simulink model "full_maneuver_platoon_new_strategy"  (R2019a)
settings: Solver=VariableStepAuto  StartTime=0.0  StopTime=70  FixedStep=0.1  MaxStep=0.05  RelTol=1e-3
libraries: simulink x97, dspsigops x7, powerlib_meascontrol x7, autolibshared x7
(part 3 of 7)

== system full_maneuver_platoon_new_strategy/Fd/safeErrors ==
  errors : Inport
  AND : Logic  IconShape=distinctive  AllPortsSameDT=off  OutDataTypeStr=boolean
  Compare To Constant4 : simulink/Logic and Bit Operations/Compare To Constant  relop=>=  const=-0.1  OutDataTypeStr=boolean
  Demux : Demux  Outputs=2
  safetyFlag : Outport
  wires:
  Demux/2 -> AND/2
  Demux/1 -> AND/1
  AND/1 -> safetyFlag/1
  errors/1 -> Compare To Constant4/1
  Compare To Constant4/1 -> Demux/1

== system full_maneuver_platoon_new_strategy/Fd/safeErrors1 ==
  errors : Inport
  AND : Logic  IconShape=distinctive  AllPortsSameDT=off  OutDataTypeStr=boolean
  Compare To Constant4 : simulink/Logic and Bit Operations/Compare To Constant  relop=>=  const=-0.1  OutDataTypeStr=boolean
  Demux : Demux  Outputs=2
  safetyFlag : Outport
  wires:
  Compare To Constant4/1 -> Demux/1
  errors/1 -> Compare To Constant4/1
  AND/1 -> safetyFlag/1
  Demux/1 -> AND/1
  Demux/2 -> AND/2

== system full_maneuver_platoon_new_strategy/Fd/safeErrors2 ==
  errors : Inport
  AND : Logic  IconShape=distinctive  AllPortsSameDT=off  OutDataTypeStr=boolean
  Compare To Constant4 : simulink/Logic and Bit Operations/Compare To Constant  relop=>=  const=-0.1  OutDataTypeStr=boolean
  Demux : Demux  Outputs=2
  safetyFlag : Outport
  wires:
  Demux/2 -> AND/2
  Demux/1 -> AND/1
  AND/1 -> safetyFlag/1
  errors/1 -> Compare To Constant4/1
  Compare To Constant4/1 -> Demux/1

== system full_maneuver_platoon_new_strategy/Fd/steadyState ==
  u : Inport
  AND : Logic  IconShape=distinctive  AllPortsSameDT=off  OutDataTypeStr=boolean
  Abs2 : Abs
  Compare To Constant2 : simulink/Logic and Bit Operations/Compare To Constant  relop=<=  const=0.2  OutDataTypeStr=boolean
  Demux : Demux  Outputs=2
  Mux : Mux  Inputs=2
  Transport Delay2 : TransportDelay
  ssFlag : Outport
  wires:
  u/1 -> Transport Delay2/1, Mux/2
  Abs2/1 -> Compare To Constant2/1
  Demux/1 -> AND/1
  Transport Delay2/1 -> Mux/1
  AND/1 -> ssFlag/1
  Compare To Constant2/1 -> Demux/1
  Mux/1 -> Abs2/1
  Demux/2 -> AND/2

== system full_maneuver_platoon_new_strategy/Fo/Lateral Control ==
  <Y> : Inport
  <r> : Inport  Port=2
  startLaneChange : Inport  Port=3
  yRef : Inport  Port=4
  Demux2 : Demux
  Full State Observer : Subsystem
  Gain1 : Gain  Gain=Klat  Multiplication=Matrix(K*u)
  Integrator : Integrator  InitialCondition=y0
  Mux : Mux  Inputs=2
  Pad : dspsigops/Pad  padAlong=Columns  dimsToPad=1  valSrc=Specify via dialog  padVal=0  spec=Output size  padNumOutRowsSpecMethod=User-specified  numOutRows=4  padNumOutColsSpecMethod=User-specified  numOutCols=1  isVarDimsMode=off  padBeginning=0  padEnd=0  outSizeMode=User-specified  outSize=1  padSigAt=End  trunc_flag=None  roundingMode=Floor  overflowMode=off  truncOrWrapMode=Truncate  wrap_flag=None
      settings: SourceProductName=DSP System Toolbox  SourceProductBaseCode=DS
  Rate Limiter : RateLimiter  RisingSlewLimit=maxDeltaDot  FallingSlewLimit=-maxDeltaDot  SampleTimeMode=inherited
  Saturation : Saturate  UpperLimit=maxDelta  LowerLimit=-maxDelta
  Scope : Scope  NumInputPorts=4
  Scope1 : Scope
  Sum : Sum  Inputs=|+-
  Sum2 : Sum  Inputs=|+-
  Triggered Subsystem1 : Subsystem  TreatAsAtomicUnit=on
  delta : Outport
  wires:
  Rate Limiter/1 -> Full State Observer/2(delta), Scope1/1, delta/1  "delta"
  Demux2/1 -> Scope/1
  Integrator/1 -> Sum2/2, Pad/1
  Gain1/1 -> Saturation/1
  <r>/1 -> Mux/2
  Full State Observer/1(xhat) -> Sum/2, Demux2/1  "estStates"
  Sum/1 -> Gain1/1
  Pad/1 -> Sum/1
  Mux/1 -> Full State Observer/1(measuredOutputs)
  Demux2/4 -> Scope/4
  Demux2/2 -> Scope/2
  Sum2/1 -> Integrator/1
  Saturation/1 -> Rate Limiter/1
  Demux2/3 -> Scope/3
  Triggered Subsystem1/1(Out1) -> Sum2/1
  <Y>/1 -> Mux/1
  startLaneChange/1 -> Triggered Subsystem1/Trigger
  yRef/1 -> Triggered Subsystem1/1(In1)

== system full_maneuver_platoon_new_strategy/Fo/Regular Vehicle Following ==
  ego : Inport
  leader : Inport  Port=2
  lcFlag : Inport  Port=3
  Bus Selector : BusSelector  OutputSignals=X,Xdot,u
  Bus Selector1 : BusSelector  OutputSignals=X,Xdot
  Chart : Stateflow chart  BlockKeywords=__PRM__SERIALIZED__DATA__:Stateflow Chart,Stateflow Diagram  TreatAsAtomicUnit=on
  Compare To Constant : simulink/Logic and Bit Operations/Compare To Constant  relop=<  const=5*maxHeadwayError  OutDataTypeStr=boolean
  Compute Errors : Subsystem
  Mux : Mux  Inputs=2
  Rate Limiter : RateLimiter  RisingSlewLimit=maxJerk  FallingSlewLimit=minJerk  SampleTimeMode=inherited
  Rate Limiter1 : RateLimiter  RisingSlewLimit=maxComfJerk  FallingSlewLimit=minComfJerk  SampleTimeMode=inherited
  Scope2 : Scope
  Scope3 : Scope
  Switch1 : Switch  Criteria=u2 > Threshold
  Veh Following : Subsystem  TreatAsAtomicUnit=on
  Velocity Control : Subsystem  TreatAsAtomicUnit=on
  comf saturation : Saturate  UpperLimit=maxComfAccel  LowerLimit=minComfAccel
  safe saturation : Saturate  UpperLimit=maxAcceleration  LowerLimit=minAcceleration
  veh foll state : Scope
  u : Outport
  errors : Outport  Port=2
  gap : Outport  Port=3
  wires:
  Bus Selector/2 -> Compute Errors/2(vf), Velocity Control/1(velocity)  "<Xdot>"
  Bus Selector/1 -> Compute Errors/1(xf)  "<X>"
  Veh Following/1(u) -> Chart/2(uVehFoll)
  lcFlag/1 -> Compute Errors/5(lcFlag)
  Compute Errors/1(eh) -> Compare To Constant/1, Veh Following/1(eh), Mux/1
  Compare To Constant/1 -> Chart/1(leaderWithinRange), Veh Following/4(intReset), Velocity Control/3(intReset)
  ego/1 -> Bus Selector/1
  Compute Errors/3("gap ") -> gap/1
  Compute Errors/4(unsafeFlag) -> Switch1/2, Scope2/1
  Rate Limiter1/1 -> Switch1/3  "sat(u)"
  Bus Selector/3 -> Veh Following/3(realInput), Velocity Control/2(realInput)  "<u>"
  Chart/2(u) -> safe saturation/1, comf saturation/1
  Switch1/1 -> u/1, Scope3/1
  Rate Limiter/1 -> Switch1/1  "sat(u)"
  safe saturation/1 -> Rate Limiter/1
  comf saturation/1 -> Rate Limiter1/1
  Compute Errors/2(ev) -> Veh Following/2(ev), Mux/2
  Velocity Control/1(u) -> Chart/3(uVelControl)
  Bus Selector1/1 -> Compute Errors/3(xl)  "<X>"
  Mux/1 -> errors/1
  Chart/1(state) -> veh foll state/1
  leader/1 -> Bus Selector1/1
  Bus Selector1/2 -> Compute Errors/4(vl)  "<Xdot>"

== system full_maneuver_platoon_new_strategy/Fo/Triggered Subsystem ==
  Trigger : TriggerPort  VariantControl=Variant
  Constant : Constant
  Out1 : Outport  InitialOutput=0
  wires:
  Constant/1 -> Out1/1

== system full_maneuver_platoon_new_strategy/Fo/Vehicle Following During LC ==
  ego : Inport
  futureLeader : Inport  Port=2
  lcFlag : Inport  Port=3
  Enable : EnablePort
  Bus Selector : BusSelector  OutputSignals=X,Xdot,u
  Bus Selector1 : BusSelector  OutputSignals=X,Xdot
  Chart : Stateflow chart  BlockKeywords=__PRM__SERIALIZED__DATA__:Stateflow Chart,Stateflow Diagram  TreatAsAtomicUnit=on
  Compare To Constant : simulink/Logic and Bit Operations/Compare To Constant  relop=<  const=5*maxHeadwayError  OutDataTypeStr=boolean
  Compute Errors : Subsystem
  Mux : Mux  Inputs=2
  Rate Limiter : RateLimiter  RisingSlewLimit=maxJerk  FallingSlewLimit=minJerk  SampleTimeMode=inherited
  Scope3 : Scope
  Subsystem : Subsystem
  Terminator : Terminator
  Veh Following : Subsystem  TreatAsAtomicUnit=on
  Velocity Control : Subsystem  TreatAsAtomicUnit=on
  safe saturation : Saturate  UpperLimit=maxAcceleration  LowerLimit=minAcceleration
  veh foll state : Scope
  u : Outport
  errors : Outport  Port=2
  gap : Outport  Port=3
  lcDone : Outport  Port=4
  wires:
  futureLeader/1 -> Bus Selector1/1, Subsystem/2(futureLeader)
  Subsystem/1(lcDone) -> lcDone/1
  Bus Selector/2 -> Velocity Control/1(velocity), Compute Errors/2(vf)  "<Xdot>"
  Compute Errors/1(eh) -> Mux/1, Veh Following/1(eh), Compare To Constant/1
  Compute Errors/4(unsafeFlag) -> Terminator/1
  Chart/1(state) -> veh foll state/1
  Compute Errors/2(ev) -> Veh Following/2(ev), Mux/2
  Bus Selector1/1 -> Compute Errors/3(xl)  "<X>"
  Mux/1 -> errors/1
  lcFlag/1 -> Compute Errors/5(lcFlag), Subsystem/3(lcFlag)
  Bus Selector/3 -> Velocity Control/2(realInput), Veh Following/3(realInput)  "<u>"
  Rate Limiter/1 -> Scope3/1, u/1  "sat(u)"
  safe saturation/1 -> Rate Limiter/1
  Chart/2(u) -> safe saturation/1
  Velocity Control/1(u) -> Chart/3(uVelControl)
  ego/1 -> Subsystem/1(ego), Bus Selector/1
  Veh Following/1(u) -> Chart/2(uVehFoll)
  Compare To Constant/1 -> Velocity Control/3(intReset), Veh Following/4(intReset), Chart/1(leaderWithinRange)
  Bus Selector/1 -> Compute Errors/1(xf)  "<X>"
  Compute Errors/3("gap ") -> gap/1
  Bus Selector1/2 -> Compute Errors/4(vl)  "<Xdot>"

== system full_maneuver_platoon_new_strategy/Fo/Virtual Vehicle Following ==
  ego : Inport
  virtualLeader : Inport  Port=2
  lcFlag : Inport  Port=3
  Enable : EnablePort
  Bus Selector : BusSelector  OutputSignals=X,Xdot,u
  Bus Selector1 : BusSelector  OutputSignals=X,Xdot
  Chart : Stateflow chart  BlockKeywords=__PRM__SERIALIZED__DATA__:Stateflow Chart,Stateflow Diagram  TreatAsAtomicUnit=on
  Compute Errors : Subsystem
  Input Saturation : Saturate  UpperLimit=maxComfAccel  LowerLimit=minComfAccel
  Mux : Mux  Inputs=2
  Rate Limiter : RateLimiter  RisingSlewLimit=maxComfJerk  FallingSlewLimit=minComfJerk  SampleTimeMode=inherited
  Subsystem : Subsystem
  Sum6 : Sum  Inputs=|+-
  Terminator : Terminator
  Transport Delay1 : TransportDelay  DelayTime=0.01
  Velocity Control : Subsystem  TreatAsAtomicUnit=on
  Virtual Leader Following : Subsystem  TreatAsAtomicUnit=on
  vMin : Constant  Value=vMin
  u : Outport  InitialOutput=0
  virtualErrors : Outport  Port=2  OutputWhenDisabled=reset  InitialOutput=[0, 0]
  virtualGap : Outport  Port=3  OutputWhenDisabled=reset  InitialOutput=[0]
  lcStarted : Outport  Port=4
  wires:
  Subsystem/1(lcStarted) -> lcStarted/1
  Sum6/1 -> Velocity Control/2(ev), Chart/1(velDiff)
  virtualLeader/1 -> Subsystem/2(virtualLeader), Bus Selector1/1
  Rate Limiter/1 -> u/1  "virtualFoll"
  Mux/1 -> virtualErrors/1
  vMin/1 -> Sum6/1
  Compute Errors/1(eh) -> Virtual Leader Following/1(eh), Mux/1  "eh"
  Bus Selector/3 -> Virtual Leader Following/3(realInput)  "<u>"
  ego/1 -> Subsystem/1(ego), Bus Selector/1
  Transport Delay1/1 -> Velocity Control/1(intReset)
  Virtual Leader Following/1(u) -> Chart/3(uVehFoll)  "uVehFoll"
  Bus Selector/2 -> Compute Errors/2(vf), Sum6/2  "<Xdot>"
  Input Saturation/1 -> Rate Limiter/1
  Bus Selector/1 -> Compute Errors/1(xf)  "<X>"
  Compute Errors/3("gap ") -> virtualGap/1
  Chart/2(u) -> Input Saturation/1  "u"
  Compute Errors/4(unsafeFlag) -> Terminator/1
  Chart/1(state) -> Transport Delay1/1
  Bus Selector1/1 -> Compute Errors/3(xl)  "<X>"
  Velocity Control/1(Out1) -> Chart/2(uVelControl)  "uVelControl"
  Compute Errors/2(ev) -> Mux/2, Virtual Leader Following/2(ev)
  lcFlag/1 -> Compute Errors/5(lcFlag)
  Bus Selector1/2 -> Compute Errors/4(vl)  "<Xdot>"

== system full_maneuver_platoon_new_strategy/Fo/followerErrors ==
  ego : Inport
  follower : Inport  Port=2
  Bus Selector1 : BusSelector  OutputSignals=X,Xdot
  Bus Selector3 : BusSelector  OutputSignals=X,Xdot
  Mux : Mux  Inputs=2
  Sum3 : Sum  Inputs=-+|
  Terminator1 : Terminator
  gapToFollower : Subsystem
  errors : Outport
  wires:
  gapToFollower/2("gap ") -> Terminator1/1
  Sum3/1 -> Mux/2
  Bus Selector3/2 -> gapToFollower/2(vf), Sum3/1  "<Xdot>"
  follower/1 -> Bus Selector3/1
  gapToFollower/1(eh) -> Mux/1
  Bus Selector1/2 -> Sum3/2  "<Xdot>"
  Bus Selector3/1 -> gapToFollower/1(xf)  "<X>"
  ego/1 -> Bus Selector1/1
  Bus Selector1/1 -> gapToFollower/3(xl)  "<X>"
  Mux/1 -> errors/1

== system full_maneuver_platoon_new_strategy/Fo/safeErrors ==
  errors : Inport
  AND : Logic  IconShape=distinctive  AllPortsSameDT=off  OutDataTypeStr=boolean
  Compare To Constant4 : simulink/Logic and Bit Operations/Compare To Constant  relop=>=  const=-0.1  OutDataTypeStr=boolean
  Demux : Demux  Outputs=2
  safetyFlag : Outport
  wires:
  Demux/2 -> AND/2
  Demux/1 -> AND/1
  AND/1 -> safetyFlag/1
  errors/1 -> Compare To Constant4/1
  Compare To Constant4/1 -> Demux/1

== system full_maneuver_platoon_new_strategy/Fo/safeErrors1 ==
  errors : Inport
  AND : Logic  IconShape=distinctive  AllPortsSameDT=off  OutDataTypeStr=boolean
  Compare To Constant4 : simulink/Logic and Bit Operations/Compare To Constant  relop=>=  const=-0.1  OutDataTypeStr=boolean
  Demux : Demux  Outputs=2
  safetyFlag : Outport
  wires:
  Compare To Constant4/1 -> Demux/1
  errors/1 -> Compare To Constant4/1
  AND/1 -> safetyFlag/1
  Demux/1 -> AND/1
  Demux/2 -> AND/2

== system full_maneuver_platoon_new_strategy/Fo/safeErrors2 ==
  errors : Inport
  AND : Logic  IconShape=distinctive  AllPortsSameDT=off  OutDataTypeStr=boolean
  Compare To Constant4 : simulink/Logic and Bit Operations/Compare To Constant  relop=>=  const=-0.1  OutDataTypeStr=boolean
  Demux : Demux  Outputs=2
  safetyFlag : Outport
  wires:
  Demux/2 -> AND/2
  Demux/1 -> AND/1
  AND/1 -> safetyFlag/1
  errors/1 -> Compare To Constant4/1
  Compare To Constant4/1 -> Demux/1

== system full_maneuver_platoon_new_strategy/Fo/steadyState ==
  u : Inport
  AND : Logic  IconShape=distinctive  AllPortsSameDT=off  OutDataTypeStr=boolean
  Abs1 : Abs
  Abs2 : Abs
  Compare To Constant1 : simulink/Logic and Bit Operations/Compare To Constant  relop=<=  const=0.5  OutDataTypeStr=boolean
  Compare To Constant2 : simulink/Logic and Bit Operations/Compare To Constant  relop=<=  const=0.5  OutDataTypeStr=boolean
  Transport Delay2 : TransportDelay
  ssFlag : Outport
  wires:
  u/1 -> Abs2/1, Transport Delay2/1
  Abs1/1 -> Compare To Constant1/1
  Abs2/1 -> Compare To Constant2/1
  Compare To Constant1/1 -> AND/1
  Transport Delay2/1 -> Abs1/1
  AND/1 -> ssFlag/1
  Compare To Constant2/1 -> AND/2

== system full_maneuver_platoon_new_strategy/Ld/Lateral Control ==
  <Y> : Inport
  <r> : Inport  Port=2
  startLaneChange : Inport  Port=3
  yRef : Inport  Port=4
  Demux2 : Demux
  Full State Observer : Subsystem
  Gain1 : Gain  Gain=Klat  Multiplication=Matrix(K*u)
  Integrator : Integrator  InitialCondition=y0
  Mux : Mux  Inputs=2
  Pad : dspsigops/Pad  padAlong=Columns  dimsToPad=1  valSrc=Specify via dialog  padVal=0  spec=Output size  padNumOutRowsSpecMethod=User-specified  numOutRows=4  padNumOutColsSpecMethod=User-specified  numOutCols=1  isVarDimsMode=off  padBeginning=0  padEnd=0  outSizeMode=User-specified  outSize=1  padSigAt=End  trunc_flag=None  roundingMode=Floor  overflowMode=off  truncOrWrapMode=Truncate  wrap_flag=None
      settings: SourceProductName=DSP System Toolbox  SourceProductBaseCode=DS
  Rate Limiter : RateLimiter  RisingSlewLimit=maxDeltaDot  FallingSlewLimit=-maxDeltaDot  SampleTimeMode=inherited
  Saturation : Saturate  UpperLimit=maxDelta  LowerLimit=-maxDelta
  Scope : Scope  NumInputPorts=4
  Scope1 : Scope
  Sum : Sum  Inputs=|+-
  Sum2 : Sum  Inputs=|+-
  Triggered Subsystem1 : Subsystem  TreatAsAtomicUnit=on
  delta : Outport
  wires:
  Rate Limiter/1 -> Full State Observer/2(delta), Scope1/1, delta/1  "delta"
  Demux2/1 -> Scope/1
  Integrator/1 -> Sum2/2, Pad/1
  Gain1/1 -> Saturation/1
  <r>/1 -> Mux/2
  Full State Observer/1(xhat) -> Sum/2, Demux2/1  "estStates"
  Sum/1 -> Gain1/1
  Pad/1 -> Sum/1
  Mux/1 -> Full State Observer/1(measuredOutputs)
  Demux2/4 -> Scope/4
  Demux2/2 -> Scope/2
  Sum2/1 -> Integrator/1
  Saturation/1 -> Rate Limiter/1
  Demux2/3 -> Scope/3
  Triggered Subsystem1/1(Out1) -> Sum2/1
  <Y>/1 -> Mux/1
  startLaneChange/1 -> Triggered Subsystem1/Trigger
  yRef/1 -> Triggered Subsystem1/1(In1)

== system full_maneuver_platoon_new_strategy/Ld/Regular Vehicle Following ==
  ego : Inport
  leader : Inport  Port=2
  lcFlag : Inport  Port=3
  Bus Selector : BusSelector  OutputSignals=X,Xdot,u
  Bus Selector1 : BusSelector  OutputSignals=X,Xdot
  Chart : Stateflow chart  BlockKeywords=__PRM__SERIALIZED__DATA__:Stateflow Chart,Stateflow Diagram  TreatAsAtomicUnit=on
  Compare To Constant : simulink/Logic and Bit Operations/Compare To Constant  relop=<  const=5*maxHeadwayError  OutDataTypeStr=boolean
  Compute Errors : Subsystem
  Mux : Mux  Inputs=2
  Rate Limiter : RateLimiter  RisingSlewLimit=maxJerk  FallingSlewLimit=minJerk  SampleTimeMode=inherited
  Rate Limiter1 : RateLimiter  RisingSlewLimit=maxComfJerk  FallingSlewLimit=minComfJerk  SampleTimeMode=inherited
  Scope2 : Scope
  Scope3 : Scope
  Switch1 : Switch  Criteria=u2 > Threshold
  Veh Following : Subsystem  TreatAsAtomicUnit=on
  Velocity Control : Subsystem  TreatAsAtomicUnit=on
  comf saturation : Saturate  UpperLimit=maxComfAccel  LowerLimit=minComfAccel
  safe saturation : Saturate  UpperLimit=maxAcceleration  LowerLimit=minAcceleration
  veh foll state : Scope
  u : Outport
  errors : Outport  Port=2
  gap : Outport  Port=3
  wires:
  Bus Selector/2 -> Compute Errors/2(vf), Velocity Control/1(velocity)  "<Xdot>"
  Bus Selector/1 -> Compute Errors/1(xf)  "<X>"
  Veh Following/1(u) -> Chart/2(uVehFoll)
  lcFlag/1 -> Compute Errors/5(lcFlag)
  Compute Errors/1(eh) -> Compare To Constant/1, Veh Following/1(eh), Mux/1
  Compare To Constant/1 -> Chart/1(leaderWithinRange), Veh Following/4(intReset), Velocity Control/3(intReset)
  ego/1 -> Bus Selector/1
  Compute Errors/3("gap ") -> gap/1
  Compute Errors/4(unsafeFlag) -> Switch1/2, Scope2/1
  Rate Limiter1/1 -> Switch1/3  "sat(u)"
  Bus Selector/3 -> Veh Following/3(realInput), Velocity Control/2(realInput)  "<u>"
  Chart/2(u) -> safe saturation/1, comf saturation/1
  Switch1/1 -> u/1, Scope3/1
  Rate Limiter/1 -> Switch1/1  "sat(u)"
  safe saturation/1 -> Rate Limiter/1
  comf saturation/1 -> Rate Limiter1/1
  Compute Errors/2(ev) -> Veh Following/2(ev), Mux/2
  Velocity Control/1(u) -> Chart/3(uVelControl)
  Bus Selector1/1 -> Compute Errors/3(xl)  "<X>"
  Mux/1 -> errors/1
  Chart/1(state) -> veh foll state/1
  leader/1 -> Bus Selector1/1
  Bus Selector1/2 -> Compute Errors/4(vl)  "<Xdot>"

== system full_maneuver_platoon_new_strategy/Ld/Triggered Subsystem ==
  Trigger : TriggerPort  VariantControl=Variant
  Constant : Constant
  Out1 : Outport  InitialOutput=0
  wires:
  Constant/1 -> Out1/1

== system full_maneuver_platoon_new_strategy/Ld/Vehicle Following During LC ==
  ego : Inport
  futureLeader : Inport  Port=2
  lcFlag : Inport  Port=3
  Enable : EnablePort
  Bus Selector : BusSelector  OutputSignals=X,Xdot,u
  Bus Selector1 : BusSelector  OutputSignals=X,Xdot
  Chart : Stateflow chart  BlockKeywords=__PRM__SERIALIZED__DATA__:Stateflow Chart,Stateflow Diagram  TreatAsAtomicUnit=on
  Compare To Constant : simulink/Logic and Bit Operations/Compare To Constant  relop=<  const=5*maxHeadwayError  OutDataTypeStr=boolean
  Compute Errors : Subsystem
  Mux : Mux  Inputs=2
  Rate Limiter : RateLimiter  RisingSlewLimit=maxJerk  FallingSlewLimit=minJerk  SampleTimeMode=inherited
  Scope3 : Scope
  Subsystem : Subsystem
  Terminator : Terminator
  Veh Following : Subsystem  TreatAsAtomicUnit=on
  Velocity Control : Subsystem  TreatAsAtomicUnit=on
  safe saturation : Saturate  UpperLimit=maxAcceleration  LowerLimit=minAcceleration
  veh foll state : Scope
  u : Outport
  errors : Outport  Port=2
  gap : Outport  Port=3
  lcDone : Outport  Port=4
  wires:
  futureLeader/1 -> Bus Selector1/1, Subsystem/2(futureLeader)
  Subsystem/1(lcDone) -> lcDone/1
  Bus Selector/2 -> Velocity Control/1(velocity), Compute Errors/2(vf)  "<Xdot>"
  Compute Errors/1(eh) -> Mux/1, Veh Following/1(eh), Compare To Constant/1
  Compute Errors/4(unsafeFlag) -> Terminator/1
  Chart/1(state) -> veh foll state/1
  Compute Errors/2(ev) -> Veh Following/2(ev), Mux/2
  Bus Selector1/1 -> Compute Errors/3(xl)  "<X>"
  Mux/1 -> errors/1
  lcFlag/1 -> Compute Errors/5(lcFlag), Subsystem/3(lcFlag)
  Bus Selector/3 -> Velocity Control/2(realInput), Veh Following/3(realInput)  "<u>"
  Rate Limiter/1 -> Scope3/1, u/1  "sat(u)"
  safe saturation/1 -> Rate Limiter/1
  Chart/2(u) -> safe saturation/1
  Velocity Control/1(u) -> Chart/3(uVelControl)
  ego/1 -> Subsystem/1(ego), Bus Selector/1
  Veh Following/1(u) -> Chart/2(uVehFoll)
  Compare To Constant/1 -> Velocity Control/3(intReset), Veh Following/4(intReset), Chart/1(leaderWithinRange)
  Bus Selector/1 -> Compute Errors/1(xf)  "<X>"
  Compute Errors/3("gap ") -> gap/1
  Bus Selector1/2 -> Compute Errors/4(vl)  "<Xdot>"

== system full_maneuver_platoon_new_strategy/Ld/Virtual Vehicle Following ==
  ego : Inport
  virtualLeader : Inport  Port=2
  lcFlag : Inport  Port=3
  Enable : EnablePort
  Bus Selector : BusSelector  OutputSignals=X,Xdot,u
  Bus Selector1 : BusSelector  OutputSignals=X,Xdot
  Chart : Stateflow chart  BlockKeywords=__PRM__SERIALIZED__DATA__:Stateflow Chart,Stateflow Diagram  TreatAsAtomicUnit=on
  Compute Errors : Subsystem
  Input Saturation : Saturate  UpperLimit=maxComfAccel  LowerLimit=minComfAccel
  Mux : Mux  Inputs=2
  Rate Limiter : RateLimiter  RisingSlewLimit=maxComfJerk  FallingSlewLimit=minComfJerk  SampleTimeMode=inherited
  Subsystem : Subsystem
  Sum6 : Sum  Inputs=|+-
  Terminator : Terminator
  Transport Delay1 : TransportDelay  DelayTime=0.01
  Velocity Control : Subsystem  TreatAsAtomicUnit=on
  Virtual Leader Following : Subsystem  TreatAsAtomicUnit=on
  vMin : Constant  Value=vMin
  u : Outport  InitialOutput=0
  virtualErrors : Outport  Port=2  OutputWhenDisabled=reset  InitialOutput=[0, 0]
  virtualGap : Outport  Port=3  OutputWhenDisabled=reset  InitialOutput=[0]
  lcStarted : Outport  Port=4
  wires:
  Subsystem/1(lcStarted) -> lcStarted/1
  Sum6/1 -> Velocity Control/2(ev), Chart/1(velDiff)
  virtualLeader/1 -> Subsystem/2(virtualLeader), Bus Selector1/1
  Rate Limiter/1 -> u/1  "virtualFoll"
  Mux/1 -> virtualErrors/1
  vMin/1 -> Sum6/1
  Compute Errors/1(eh) -> Virtual Leader Following/1(eh), Mux/1  "eh"
  Bus Selector/3 -> Virtual Leader Following/3(realInput)  "<u>"
  ego/1 -> Subsystem/1(ego), Bus Selector/1
  Transport Delay1/1 -> Velocity Control/1(intReset)
  Virtual Leader Following/1(u) -> Chart/3(uVehFoll)  "uVehFoll"
  Bus Selector/2 -> Compute Errors/2(vf), Sum6/2  "<Xdot>"
  Input Saturation/1 -> Rate Limiter/1
  Bus Selector/1 -> Compute Errors/1(xf)  "<X>"
  Compute Errors/3("gap ") -> virtualGap/1
  Chart/2(u) -> Input Saturation/1  "u"
  Compute Errors/4(unsafeFlag) -> Terminator/1
  Chart/1(state) -> Transport Delay1/1
  Bus Selector1/1 -> Compute Errors/3(xl)  "<X>"
  Velocity Control/1(Out1) -> Chart/2(uVelControl)  "uVelControl"
  Compute Errors/2(ev) -> Mux/2, Virtual Leader Following/2(ev)
  lcFlag/1 -> Compute Errors/5(lcFlag)
  Bus Selector1/2 -> Compute Errors/4(vl)  "<Xdot>"

== system full_maneuver_platoon_new_strategy/Ld/followerErrors ==
  ego : Inport
  follower : Inport  Port=2
  Bus Selector1 : BusSelector  OutputSignals=X,Xdot
  Bus Selector3 : BusSelector  OutputSignals=X,Xdot
  Mux : Mux  Inputs=2
  Sum3 : Sum  Inputs=-+|
  Terminator1 : Terminator
  gapToFollower : Subsystem
  errors : Outport
  wires:
  gapToFollower/2("gap ") -> Terminator1/1
  Sum3/1 -> Mux/2
  Bus Selector3/2 -> gapToFollower/2(vf), Sum3/1  "<Xdot>"
  follower/1 -> Bus Selector3/1
  gapToFollower/1(eh) -> Mux/1
  Bus Selector1/2 -> Sum3/2  "<Xdot>"
  Bus Selector3/1 -> gapToFollower/1(xf)  "<X>"
  ego/1 -> Bus Selector1/1
  Bus Selector1/1 -> gapToFollower/3(xl)  "<X>"
  Mux/1 -> errors/1

== system full_maneuver_platoon_new_strategy/Ld/safeErrors ==
  errors : Inport
  AND : Logic  IconShape=distinctive  AllPortsSameDT=off  OutDataTypeStr=boolean
  Compare To Constant4 : simulink/Logic and Bit Operations/Compare To Constant  relop=>=  const=-0.1  OutDataTypeStr=boolean
  Demux : Demux  Outputs=2
  safetyFlag : Outport
  wires:
  Demux/2 -> AND/2
  Demux/1 -> AND/1
  AND/1 -> safetyFlag/1
  errors/1 -> Compare To Constant4/1
  Compare To Constant4/1 -> Demux/1

== system full_maneuver_platoon_new_strategy/Ld/safeErrors1 ==
  errors : Inport
  AND : Logic  IconShape=distinctive  AllPortsSameDT=off  OutDataTypeStr=boolean
  Compare To Constant4 : simulink/Logic and Bit Operations/Compare To Constant  relop=>=  const=-0.1  OutDataTypeStr=boolean
  Demux : Demux  Outputs=2
  safetyFlag : Outport
  wires:
  Compare To Constant4/1 -> Demux/1
  errors/1 -> Compare To Constant4/1
  AND/1 -> safetyFlag/1
  Demux/1 -> AND/1
  Demux/2 -> AND/2

== system full_maneuver_platoon_new_strategy/Ld/safeErrors2 ==
  errors : Inport
  AND : Logic  IconShape=distinctive  AllPortsSameDT=off  OutDataTypeStr=boolean
  Compare To Constant4 : simulink/Logic and Bit Operations/Compare To Constant  relop=>=  const=-0.1  OutDataTypeStr=boolean
  Demux : Demux  Outputs=2
  safetyFlag : Outport
  wires:
  Demux/2 -> AND/2
  Demux/1 -> AND/1
  AND/1 -> safetyFlag/1
  errors/1 -> Compare To Constant4/1
  Compare To Constant4/1 -> Demux/1

== system full_maneuver_platoon_new_strategy/Ld/steadyState ==
  u : Inport
  AND : Logic  IconShape=distinctive  AllPortsSameDT=off  OutDataTypeStr=boolean
  Abs1 : Abs
  Abs2 : Abs
  Compare To Constant1 : simulink/Logic and Bit Operations/Compare To Constant  relop=<=  const=0.5  OutDataTypeStr=boolean
  Compare To Constant2 : simulink/Logic and Bit Operations/Compare To Constant  relop=<=  const=0.5  OutDataTypeStr=boolean
  Transport Delay2 : TransportDelay
  ssFlag : Outport
  wires:
  u/1 -> Abs2/1, Transport Delay2/1
  Abs1/1 -> Compare To Constant1/1
  Abs2/1 -> Compare To Constant2/1
  Compare To Constant1/1 -> AND/1
  Transport Delay2/1 -> Abs1/1
  AND/1 -> ssFlag/1
  Compare To Constant2/1 -> AND/2

== system full_maneuver_platoon_new_strategy/Lo/Lateral Control ==
  <Y> : Inport
  <r> : Inport  Port=2
  startLaneChange : Inport  Port=3
  yRef : Inport  Port=4
  Demux2 : Demux
  Full State Observer : Subsystem
  Gain1 : Gain  Gain=Klat  Multiplication=Matrix(K*u)
  Integrator : Integrator  InitialCondition=y0
  Mux : Mux  Inputs=2
  Pad : dspsigops/Pad  padAlong=Columns  dimsToPad=1  valSrc=Specify via dialog  padVal=0  spec=Output size  padNumOutRowsSpecMethod=User-specified  numOutRows=4  padNumOutColsSpecMethod=User-specified  numOutCols=1  isVarDimsMode=off  padBeginning=0  padEnd=0  outSizeMode=User-specified  outSize=1  padSigAt=End  trunc_flag=None  roundingMode=Floor  overflowMode=off  truncOrWrapMode=Truncate  wrap_flag=None
      settings: SourceProductName=DSP System Toolbox  SourceProductBaseCode=DS
  Rate Limiter : RateLimiter  RisingSlewLimit=maxDeltaDot  FallingSlewLimit=-maxDeltaDot  SampleTimeMode=inherited
  Saturation : Saturate  UpperLimit=maxDelta  LowerLimit=-maxDelta
  Scope : Scope  NumInputPorts=4
  Scope1 : Scope
  Sum : Sum  Inputs=|+-
  Sum2 : Sum  Inputs=|+-
  Triggered Subsystem1 : Subsystem  TreatAsAtomicUnit=on
  delta : Outport
  wires:
  yRef/1 -> Triggered Subsystem1/1(In1)
  startLaneChange/1 -> Triggered Subsystem1/Trigger
  <Y>/1 -> Mux/1
  Triggered Subsystem1/1(Out1) -> Sum2/1
  Demux2/3 -> Scope/3
  Saturation/1 -> Rate Limiter/1
  Sum2/1 -> Integrator/1
  Demux2/2 -> Scope/2
  Demux2/4 -> Scope/4
  Mux/1 -> Full State Observer/1(measuredOutputs)
  Pad/1 -> Sum/1
  Sum/1 -> Gain1/1
  Full State Observer/1(xhat) -> Demux2/1, Sum/2  "estStates"
  <r>/1 -> Mux/2
  Gain1/1 -> Saturation/1
  Integrator/1 -> Pad/1, Sum2/2
  Demux2/1 -> Scope/1
  Rate Limiter/1 -> delta/1, Scope1/1, Full State Observer/2(delta)  "delta"

== system full_maneuver_platoon_new_strategy/Lo/Regular Vehicle Following ==
  ego : Inport
  leader : Inport  Port=2
  lcFlag : Inport  Port=3
  Bus Selector : BusSelector  OutputSignals=X,Xdot,u
  Bus Selector1 : BusSelector  OutputSignals=X,Xdot
  Chart : Stateflow chart  BlockKeywords=__PRM__SERIALIZED__DATA__:Stateflow Chart,Stateflow Diagram  TreatAsAtomicUnit=on
  Compare To Constant : simulink/Logic and Bit Operations/Compare To Constant  relop=<  const=5*maxHeadwayError  OutDataTypeStr=boolean
  Compute Errors : Subsystem
  Mux : Mux  Inputs=2
  Rate Limiter : RateLimiter  RisingSlewLimit=maxJerk  FallingSlewLimit=minJerk  SampleTimeMode=inherited
  Rate Limiter1 : RateLimiter  RisingSlewLimit=maxComfJerk  FallingSlewLimit=minComfJerk  SampleTimeMode=inherited
  Scope2 : Scope
  Scope3 : Scope
  Switch1 : Switch  Criteria=u2 > Threshold
  Veh Following : Subsystem  TreatAsAtomicUnit=on
  Velocity Control : Subsystem  TreatAsAtomicUnit=on
  comf saturation : Saturate  UpperLimit=maxComfAccel  LowerLimit=minComfAccel
  safe saturation : Saturate  UpperLimit=maxAcceleration  LowerLimit=minAcceleration
  veh foll state : Scope
  u : Outport
  errors : Outport  Port=2
  gap : Outport  Port=3
  wires:
  Bus Selector1/2 -> Compute Errors/4(vl)  "<Xdot>"
  leader/1 -> Bus Selector1/1
  Chart/1(state) -> veh foll state/1
  Mux/1 -> errors/1
  Bus Selector1/1 -> Compute Errors/3(xl)  "<X>"
  Velocity Control/1(u) -> Chart/3(uVelControl)
  Compute Errors/2(ev) -> Mux/2, Veh Following/2(ev)
  comf saturation/1 -> Rate Limiter1/1
  safe saturation/1 -> Rate Limiter/1
  Rate Limiter/1 -> Switch1/1  "sat(u)"
  Switch1/1 -> Scope3/1, u/1
  Chart/2(u) -> comf saturation/1, safe saturation/1
  Bus Selector/3 -> Velocity Control/2(realInput), Veh Following/3(realInput)  "<u>"
  Rate Limiter1/1 -> Switch1/3  "sat(u)"
  Compute Errors/4(unsafeFlag) -> Scope2/1, Switch1/2
  Compute Errors/3("gap ") -> gap/1
  ego/1 -> Bus Selector/1
  Compare To Constant/1 -> Velocity Control/3(intReset), Veh Following/4(intReset), Chart/1(leaderWithinRange)
  Compute Errors/1(eh) -> Mux/1, Veh Following/1(eh), Compare To Constant/1
  lcFlag/1 -> Compute Errors/5(lcFlag)
  Veh Following/1(u) -> Chart/2(uVehFoll)
  Bus Selector/1 -> Compute Errors/1(xf)  "<X>"
  Bus Selector/2 -> Velocity Control/1(velocity), Compute Errors/2(vf)  "<Xdot>"

== system full_maneuver_platoon_new_strategy/Lo/Triggered Subsystem ==
  Trigger : TriggerPort  VariantControl=Variant
  Constant : Constant
  Out1 : Outport  InitialOutput=0
  wires:
  Constant/1 -> Out1/1

== system full_maneuver_platoon_new_strategy/Lo/Vehicle Following During LC ==
  ego : Inport
  futureLeader : Inport  Port=2
  lcFlag : Inport  Port=3
  Enable : EnablePort
  Bus Selector : BusSelector  OutputSignals=X,Xdot,u
  Bus Selector1 : BusSelector  OutputSignals=X,Xdot
  Chart : Stateflow chart  BlockKeywords=__PRM__SERIALIZED__DATA__:Stateflow Chart,Stateflow Diagram  TreatAsAtomicUnit=on
  Compare To Constant : simulink/Logic and Bit Operations/Compare To Constant  relop=<  const=5*maxHeadwayError  OutDataTypeStr=boolean
  Compute Errors : Subsystem
  Mux : Mux  Inputs=2
  Rate Limiter : RateLimiter  RisingSlewLimit=maxJerk  FallingSlewLimit=minJerk  SampleTimeMode=inherited
  Scope3 : Scope
  Subsystem : Subsystem
  Terminator : Terminator
  Veh Following : Subsystem  TreatAsAtomicUnit=on
  Velocity Control : Subsystem  TreatAsAtomicUnit=on
  safe saturation : Saturate  UpperLimit=maxAcceleration  LowerLimit=minAcceleration
  veh foll state : Scope
  u : Outport
  errors : Outport  Port=2
  gap : Outport  Port=3
  lcDone : Outport  Port=4
  wires:
  Bus Selector1/2 -> Compute Errors/4(vl)  "<Xdot>"
  Compute Errors/3("gap ") -> gap/1
  Bus Selector/1 -> Compute Errors/1(xf)  "<X>"
  Compare To Constant/1 -> Chart/1(leaderWithinRange), Veh Following/4(intReset), Velocity Control/3(intReset)
  Veh Following/1(u) -> Chart/2(uVehFoll)
  ego/1 -> Bus Selector/1, Subsystem/1(ego)
  Velocity Control/1(u) -> Chart/3(uVelControl)
  Chart/2(u) -> safe saturation/1
  safe saturation/1 -> Rate Limiter/1
  Rate Limiter/1 -> u/1, Scope3/1  "sat(u)"
  Bus Selector/3 -> Veh Following/3(realInput), Velocity Control/2(realInput)  "<u>"
  lcFlag/1 -> Subsystem/3(lcFlag), Compute Errors/5(lcFlag)
  Mux/1 -> errors/1
  Bus Selector1/1 -> Compute Errors/3(xl)  "<X>"
  Compute Errors/2(ev) -> Mux/2, Veh Following/2(ev)
  Chart/1(state) -> veh foll state/1
  Compute Errors/4(unsafeFlag) -> Terminator/1
  Compute Errors/1(eh) -> Compare To Constant/1, Veh Following/1(eh), Mux/1
  Bus Selector/2 -> Compute Errors/2(vf), Velocity Control/1(velocity)  "<Xdot>"
  Subsystem/1(lcDone) -> lcDone/1
  futureLeader/1 -> Subsystem/2(futureLeader), Bus Selector1/1

== system full_maneuver_platoon_new_strategy/Lo/Virtual Vehicle Following ==
  ego : Inport
  virtualLeader : Inport  Port=2
  lcFlag : Inport  Port=3
  Enable : EnablePort
  Bus Selector : BusSelector  OutputSignals=X,Xdot,u
  Bus Selector1 : BusSelector  OutputSignals=X,Xdot
  Chart : Stateflow chart  BlockKeywords=__PRM__SERIALIZED__DATA__:Stateflow Chart,Stateflow Diagram  TreatAsAtomicUnit=on
  Compute Errors : Subsystem
  Input Saturation : Saturate  UpperLimit=maxComfAccel  LowerLimit=minComfAccel
  Mux : Mux  Inputs=2
  Rate Limiter : RateLimiter  RisingSlewLimit=maxComfJerk  FallingSlewLimit=minComfJerk  SampleTimeMode=inherited
  Subsystem : Subsystem
  Sum6 : Sum  Inputs=|+-
  Terminator : Terminator
  Transport Delay1 : TransportDelay  DelayTime=0.01
  Velocity Control : Subsystem  TreatAsAtomicUnit=on
  Virtual Leader Following : Subsystem  TreatAsAtomicUnit=on
  vMin : Constant  Value=vMin
  u : Outport  InitialOutput=0
  virtualErrors : Outport  Port=2  OutputWhenDisabled=reset  InitialOutput=[0, 0]
  virtualGap : Outport  Port=3  OutputWhenDisabled=reset  InitialOutput=[0]
  lcStarted : Outport  Port=4
  wires:
  Bus Selector1/2 -> Compute Errors/4(vl)  "<Xdot>"
  lcFlag/1 -> Compute Errors/5(lcFlag)
  Compute Errors/2(ev) -> Virtual Leader Following/2(ev), Mux/2
  Velocity Control/1(Out1) -> Chart/2(uVelControl)  "uVelControl"
  Bus Selector1/1 -> Compute Errors/3(xl)  "<X>"
  Chart/1(state) -> Transport Delay1/1
  Compute Errors/4(unsafeFlag) -> Terminator/1
  Chart/2(u) -> Input Saturation/1  "u"
  Compute Errors/3("gap ") -> virtualGap/1
  Bus Selector/1 -> Compute Errors/1(xf)  "<X>"
  Input Saturation/1 -> Rate Limiter/1
  Bus Selector/2 -> Sum6/2, Compute Errors/2(vf)  "<Xdot>"
  Virtual Leader Following/1(u) -> Chart/3(uVehFoll)  "uVehFoll"
  Transport Delay1/1 -> Velocity Control/1(intReset)
  ego/1 -> Bus Selector/1, Subsystem/1(ego)
  Bus Selector/3 -> Virtual Leader Following/3(realInput)  "<u>"
  Compute Errors/1(eh) -> Mux/1, Virtual Leader Following/1(eh)  "eh"
  vMin/1 -> Sum6/1
  Mux/1 -> virtualErrors/1
  Rate Limiter/1 -> u/1  "virtualFoll"
  virtualLeader/1 -> Bus Selector1/1, Subsystem/2(virtualLeader)
  Sum6/1 -> Chart/1(velDiff), Velocity Control/2(ev)
  Subsystem/1(lcStarted) -> lcStarted/1

== system full_maneuver_platoon_new_strategy/Lo/followerErrors ==
  ego : Inport
  follower : Inport  Port=2
  Bus Selector1 : BusSelector  OutputSignals=X,Xdot
  Bus Selector3 : BusSelector  OutputSignals=X,Xdot
  Mux : Mux  Inputs=2
  Sum3 : Sum  Inputs=-+|
  Terminator1 : Terminator
  gapToFollower : Subsystem
  errors : Outport
  wires:
  Mux/1 -> errors/1
  Bus Selector1/1 -> gapToFollower/3(xl)  "<X>"
  ego/1 -> Bus Selector1/1
  Bus Selector3/1 -> gapToFollower/1(xf)  "<X>"
  Bus Selector1/2 -> Sum3/2  "<Xdot>"
  gapToFollower/1(eh) -> Mux/1
  follower/1 -> Bus Selector3/1
  Bus Selector3/2 -> Sum3/1, gapToFollower/2(vf)  "<Xdot>"
  Sum3/1 -> Mux/2
  gapToFollower/2("gap ") -> Terminator1/1

== system full_maneuver_platoon_new_strategy/Lo/safeErrors ==
  errors : Inport
  AND : Logic  IconShape=distinctive  AllPortsSameDT=off  OutDataTypeStr=boolean
  Compare To Constant4 : simulink/Logic and Bit Operations/Compare To Constant  relop=>=  const=-0.1  OutDataTypeStr=boolean
  Demux : Demux  Outputs=2
  safetyFlag : Outport
  wires:
  Compare To Constant4/1 -> Demux/1
  errors/1 -> Compare To Constant4/1
  AND/1 -> safetyFlag/1
  Demux/1 -> AND/1
  Demux/2 -> AND/2

== system full_maneuver_platoon_new_strategy/Lo/safeErrors1 ==
  errors : Inport
  AND : Logic  IconShape=distinctive  AllPortsSameDT=off  OutDataTypeStr=boolean
  Compare To Constant4 : simulink/Logic and Bit Operations/Compare To Constant  relop=>=  const=-0.1  OutDataTypeStr=boolean
  Demux : Demux  Outputs=2
  safetyFlag : Outport
  wires:
  Demux/2 -> AND/2
  Demux/1 -> AND/1
  AND/1 -> safetyFlag/1
  errors/1 -> Compare To Constant4/1
  Compare To Constant4/1 -> Demux/1

== system full_maneuver_platoon_new_strategy/Lo/safeErrors2 ==
  errors : Inport
  AND : Logic  IconShape=distinctive  AllPortsSameDT=off  OutDataTypeStr=boolean
  Compare To Constant4 : simulink/Logic and Bit Operations/Compare To Constant  relop=>=  const=-0.1  OutDataTypeStr=boolean
  Demux : Demux  Outputs=2
  safetyFlag : Outport
  wires:
  Compare To Constant4/1 -> Demux/1
  errors/1 -> Compare To Constant4/1
  AND/1 -> safetyFlag/1
  Demux/1 -> AND/1
  Demux/2 -> AND/2

== system full_maneuver_platoon_new_strategy/Lo/steadyState ==
  u : Inport
  AND : Logic  IconShape=distinctive  AllPortsSameDT=off  OutDataTypeStr=boolean
  Abs1 : Abs
  Abs2 : Abs
  Compare To Constant1 : simulink/Logic and Bit Operations/Compare To Constant  relop=<=  const=0.5  OutDataTypeStr=boolean
  Compare To Constant2 : simulink/Logic and Bit Operations/Compare To Constant  relop=<=  const=0.5  OutDataTypeStr=boolean
  Transport Delay2 : TransportDelay
  ssFlag : Outport
  wires:
  Compare To Constant2/1 -> AND/2
  AND/1 -> ssFlag/1
  Transport Delay2/1 -> Abs1/1
  Compare To Constant1/1 -> AND/1
  Abs2/1 -> Compare To Constant2/1
  Abs1/1 -> Compare To Constant1/1
  u/1 -> Transport Delay2/1, Abs2/1

== system full_maneuver_platoon_new_strategy/p1/Lateral Control ==
  <Y> : Inport
  <r> : Inport  Port=2
  startLaneChange : Inport  Port=3
  yRef : Inport  Port=4
  Demux2 : Demux
  Full State Observer : Subsystem
  Gain1 : Gain  Gain=Klat  Multiplication=Matrix(K*u)
  Integrator : Integrator  InitialCondition=y0
  Mux : Mux  Inputs=2
  Pad : dspsigops/Pad  padAlong=Columns  dimsToPad=1  valSrc=Specify via dialog  padVal=0  spec=Output size  padNumOutRowsSpecMethod=User-specified  numOutRows=4  padNumOutColsSpecMethod=User-specified  numOutCols=1  isVarDimsMode=off  padBeginning=0  padEnd=0  outSizeMode=User-specified  outSize=1  padSigAt=End  trunc_flag=None  roundingMode=Floor  overflowMode=off  truncOrWrapMode=Truncate  wrap_flag=None
      settings: SourceProductName=DSP System Toolbox  SourceProductBaseCode=DS
  Rate Limiter : RateLimiter  RisingSlewLimit=maxDeltaDot  FallingSlewLimit=-maxDeltaDot  SampleTimeMode=inherited
  Saturation : Saturate  UpperLimit=maxDelta  LowerLimit=-maxDelta
  Scope : Scope  NumInputPorts=4
  Scope1 : Scope
  Sum : Sum  Inputs=|+-
  Sum2 : Sum  Inputs=|+-
  Triggered Subsystem1 : Subsystem  TreatAsAtomicUnit=on
  delta : Outport
  wires:
  yRef/1 -> Triggered Subsystem1/1(In1)
  startLaneChange/1 -> Triggered Subsystem1/Trigger
  <Y>/1 -> Mux/1
  Triggered Subsystem1/1(Out1) -> Sum2/1
  Demux2/3 -> Scope/3
  Saturation/1 -> Rate Limiter/1
  Sum2/1 -> Integrator/1
  Demux2/2 -> Scope/2
  Demux2/4 -> Scope/4
  Mux/1 -> Full State Observer/1(measuredOutputs)
  Pad/1 -> Sum/1
  Sum/1 -> Gain1/1
  Full State Observer/1(xhat) -> Demux2/1, Sum/2  "estStates"
  <r>/1 -> Mux/2
  Gain1/1 -> Saturation/1
  Integrator/1 -> Pad/1, Sum2/2
  Demux2/1 -> Scope/1
  Rate Limiter/1 -> delta/1, Scope1/1, Full State Observer/2(delta)  "delta"

== system full_maneuver_platoon_new_strategy/p1/Regular Vehicle Following ==
  ego : Inport
  leader : Inport  Port=2
  extraSpaceFlag : Inport  Port=3
  Bus Selector : BusSelector  OutputSignals=X,Xdot,u
  Bus Selector1 : BusSelector  OutputSignals=X,Xdot
  Chart : Stateflow chart  BlockKeywords=__PRM__SERIALIZED__DATA__:Stateflow Chart,Stateflow Diagram  TreatAsAtomicUnit=on
  Compare To Constant : simulink/Logic and Bit Operations/Compare To Constant  relop=<  const=5*maxHeadwayError  OutDataTypeStr=boolean
  Compute Errors : Subsystem
  Mux : Mux  Inputs=2
  Rate Limiter : RateLimiter  RisingSlewLimit=maxJerk  FallingSlewLimit=minJerk  SampleTimeMode=inherited
  Rate Limiter1 : RateLimiter  RisingSlewLimit=maxComfJerk  FallingSlewLimit=minComfJerk  SampleTimeMode=inherited
  Scope2 : Scope
  Switch1 : Switch  Criteria=u2 > Threshold
  Veh Following : Subsystem  TreatAsAtomicUnit=on
  Velocity Control : Subsystem  TreatAsAtomicUnit=on
  comf saturation : Saturate  UpperLimit=maxComfAccel  LowerLimit=minComfAccel
  eh : Scope
  output : Scope
  safe saturation : Saturate  UpperLimit=maxAcceleration  LowerLimit=minAcceleration
  veh foll state : Scope  NumInputPorts=2
  u : Outport
  errors : Outport  Port=2
  gap : Outport  Port=3
  leaderInRange : Outport  Port=4
  wires:
  Bus Selector1/2 -> Compute Errors/4(vl)  "<Xdot>"
  leader/1 -> Bus Selector1/1
  Chart/1(state) -> veh foll state/1
  Mux/1 -> errors/1
  Bus Selector1/1 -> Compute Errors/3(xl)  "<X>"
  Velocity Control/1(u) -> Chart/3(uVelControl)
  Compute Errors/2(ev) -> Mux/2, Veh Following/2(ev)
  comf saturation/1 -> Rate Limiter1/1
  safe saturation/1 -> Rate Limiter/1
  Rate Limiter/1 -> Switch1/1  "sat(u)"
  Switch1/1 -> output/1, u/1
  Chart/2(u) -> comf saturation/1, safe saturation/1, veh foll state/2
  Bus Selector/3 -> Velocity Control/2(realInput), Veh Following/3(realInput)  "<u>"
  Rate Limiter1/1 -> Switch1/3  "sat(u)"
  Compute Errors/4(unsafeFlag) -> Scope2/1, Switch1/2
  Compute Errors/3("gap ") -> gap/1
  ego/1 -> Bus Selector/1
  Compare To Constant/1 -> Velocity Control/3(intReset), Veh Following/4(intReset), Chart/1(leaderWithinRange), leaderInRange/1
  Compute Errors/1(eh) -> Mux/1, Veh Following/1(eh), Compare To Constant/1, eh/1
  extraSpaceFlag/1 -> Compute Errors/5(extraSpaceFlag)
  Veh Following/1(u) -> Chart/2(uVehFoll)
  Bus Selector/1 -> Compute Errors/1(xf)  "<X>"
  Bus Selector/2 -> Velocity Control/1(velocity), Compute Errors/2(vf)  "<Xdot>"

== system full_maneuver_platoon_new_strategy/p1/Subsystem ==
  note: Condition for Gap Generating Vehicle
  note: Condition for Lane Changing Vehicle
  lcFlag : Inport
  ego : Inport  Port=2  OutDataTypeStr=Bus: vehStatesBus
  virtualLeader : Inport  Port=3  OutDataTypeStr=Bus: vehStatesBus
  lcCanStart : Inport  Port=4
  AND : Logic  IconShape=distinctive  AllPortsSameDT=off  OutDataTypeStr=boolean
  AND1 : Logic  IconShape=distinctive  AllPortsSameDT=off  OutDataTypeStr=boolean
  Abs : Abs
  Bus Selector : BusSelector  OutputSignals=Y
  Bus Selector1 : BusSelector  OutputSignals=Y
  Compare To Constant : simulink/Logic and Bit Operations/Compare To Constant  relop=<  const=3.6-0.5  OutDataTypeStr=boolean
  NOT : Logic  Operator=NOT  IconShape=distinctive  AllPortsSameDT=off  OutDataTypeStr=boolean
  OR : Logic  Operator=OR  IconShape=distinctive  AllPortsSameDT=off  OutDataTypeStr=boolean
  Scope : Scope  NumInputPorts=3
  Sum : Sum  Inputs=+-
  lcStarted : Outport
  wires:
  AND/1 -> OR/2
  AND1/1 -> OR/1
  OR/1 -> lcStarted/1
  NOT/1 -> AND1/2
  lcCanStart/1 -> AND/2
  lcFlag/1 -> AND/1, NOT/1
  Abs/1 -> Compare To Constant/1, Scope/3
  Sum/1 -> Abs/1
  Compare To Constant/1 -> AND1/1
  Bus Selector1/1 -> Sum/2, Scope/2  "<Y>"
  Bus Selector/1 -> Sum/1, Scope/1  "<Y>"
  virtualLeader/1 -> Bus Selector1/1
  ego/1 -> Bus Selector/1

== system full_maneuver_platoon_new_strategy/p1/Subsystem1 ==
  note: Condition for Gap
      | Generating Vehicle
  note: Condition for Lane
      | Changing Vehicle
  ego : Inport  OutDataTypeStr=Bus: vehStatesBus
  futureLeader : Inport  Port=2  OutDataTypeStr=Bus: vehStatesBus
  lcFlag : Inport  Port=3
  AND : Logic  IconShape=distinctive  AllPortsSameDT=off  OutDataTypeStr=boolean
  AND1 : Logic  IconShape=distinctive  AllPortsSameDT=off  OutDataTypeStr=boolean
  Abs : Abs
  Bus Selector1 : BusSelector  OutputSignals=Y
  Bus Selector2 : BusSelector  OutputSignals=Y
  Compare To Constant : simulink/Logic and Bit Operations/Compare To Constant  relop=<=  const=1.8  OutDataTypeStr=boolean
  Compare To Constant1 : simulink/Logic and Bit Operations/Compare To Constant  relop=<=  const=0.5  OutDataTypeStr=boolean
  NOT : Logic  Operator=NOT  IconShape=distinctive  AllPortsSameDT=off  OutDataTypeStr=boolean
  OR : Logic  Operator=OR  IconShape=distinctive  AllPortsSameDT=off  OutDataTypeStr=boolean
  Scope : Scope  NumInputPorts=2
  Sum1 : Sum  Inputs=|+-
  lcDone : Outport
  wires:
  NOT/1 -> AND/2
  Abs/1 -> Compare To Constant/1, Compare To Constant1/1
  Bus Selector2/1 -> Sum1/1  "<Y>"
  AND1/1 -> OR/2, Scope/2
  OR/1 -> lcDone/1
  Compare To Constant1/1 -> AND1/1
  Sum1/1 -> Abs/1
  ego/1 -> Bus Selector2/1
  lcFlag/1 -> NOT/1, AND1/2
  Compare To Constant/1 -> AND/1
  AND/1 -> OR/1, Scope/1
  Bus Selector1/1 -> Sum1/2  "<Y>"
  futureLeader/1 -> Bus Selector1/1

== system full_maneuver_platoon_new_strategy/p1/Triggered Subsystem ==
  Trigger : TriggerPort  VariantControl=Variant
  Constant : Constant
  Out1 : Outport  InitialOutput=0
  wires:
  Constant/1 -> Out1/1

== system full_maneuver_platoon_new_strategy/p1/Triggered Subsystem1 ==
  Trigger : TriggerPort  VariantControl=Variant
  Constant : Constant
  Out1 : Outport  InitialOutput=0
  wires:
  Constant/1 -> Out1/1

== system full_maneuver_platoon_new_strategy/p1/Vehicle Following During LC ==
  ego : Inport
  futureLeader : Inport  Port=2
  extraSpaceFlag : Inport  Port=3
  Enable : EnablePort
  Bus Selector : BusSelector  OutputSignals=X,Xdot,u
  Bus Selector1 : BusSelector  OutputSignals=X,Xdot
  Chart : Stateflow chart  BlockKeywords=__PRM__SERIALIZED__DATA__:Stateflow Chart,Stateflow Diagram  TreatAsAtomicUnit=on
  Compare To Constant : simulink/Logic and Bit Operations/Compare To Constant  relop=<  const=5*maxHeadwayError  OutDataTypeStr=boolean
  Compute Errors : Subsystem
  Mux : Mux  Inputs=2
  Scope : Scope
  Scope3 : Scope
  Terminator : Terminator
  Veh Following : Subsystem  TreatAsAtomicUnit=on
  Velocity Control : Subsystem  TreatAsAtomicUnit=on
  safe acceleration : Saturate  UpperLimit=maxAcceleration  LowerLimit=minAcceleration
  safe jerk : RateLimiter  RisingSlewLimit=maxJerk  FallingSlewLimit=minJerk  SampleTimeMode=inherited
  veh foll state : Scope
  u : Outport  InitialOutput=0
  errors : Outport  Port=2
  gap : Outport  Port=3
  wires:
  Bus Selector1/2 -> Compute Errors/4(vl)  "<Xdot>"
  Compute Errors/3("gap ") -> gap/1
  Bus Selector/1 -> Compute Errors/1(xf)  "<X>"
  Compare To Constant/1 -> Chart/1(leaderWithinRange), Veh Following/4(intReset), Velocity Control/3(intReset)
  Veh Following/1(u) -> Chart/2(uVehFoll)
  ego/1 -> Bus Selector/1
  Velocity Control/1(u) -> Chart/3(uVelControl)
  Chart/2(u) -> safe acceleration/1
  safe acceleration/1 -> safe jerk/1
  safe jerk/1 -> u/1, Scope3/1  "sat(u)"
  Bus Selector/3 -> Veh Following/3(realInput), Velocity Control/2(realInput)  "<u>"
  extraSpaceFlag/1 -> Compute Errors/5(extraSpaceFlag)
  Mux/1 -> errors/1
  Bus Selector1/1 -> Compute Errors/3(xl)  "<X>"
  Compute Errors/2(ev) -> Mux/2, Veh Following/2(ev)
  Chart/1(state) -> veh foll state/1
  Compute Errors/4(unsafeFlag) -> Terminator/1
  Compute Errors/1(eh) -> Compare To Constant/1, Scope/1, Veh Following/1(eh), Mux/1
  Bus Selector/2 -> Compute Errors/2(vf), Velocity Control/1(velocity)  "<Xdot>"
  futureLeader/1 -> Bus Selector1/1

== system full_maneuver_platoon_new_strategy/p1/Virtual Vehicle Following ==
  ego : Inport
  virtualLeader : Inport  Port=2
  extraSpaceFlag : Inport  Port=3
  Enable : EnablePort
  Bus Selector : BusSelector  OutputSignals=X,Xdot,u
  Bus Selector1 : BusSelector  OutputSignals=X,Xdot
  Chart : Stateflow chart  BlockKeywords=__PRM__SERIALIZED__DATA__:Stateflow Chart,Stateflow Diagram  TreatAsAtomicUnit=on
  Compute Errors : Subsystem
  Mux : Mux  Inputs=2
  Scope : Scope
  Sum6 : Sum  Inputs=|+-
  Terminator : Terminator
  Transport Delay1 : TransportDelay  DelayTime=0.01
  Velocity Control : Subsystem  TreatAsAtomicUnit=on
  Virtual Leader Following : Subsystem  TreatAsAtomicUnit=on
  accel saturation : Saturate  UpperLimit=maxComfAccel  LowerLimit=minComfAccel
  jerk saturation : RateLimiter  RisingSlewLimit=maxComfJerk  FallingSlewLimit=minComfJerk  SampleTimeMode=inherited
  vMin : Constant  Value=vMin
  u : Outport  InitialOutput=0
  virtualErrors : Outport  Port=2  OutputWhenDisabled=reset  InitialOutput=[0, 0]
  virtualGap : Outport  Port=3  OutputWhenDisabled=reset  InitialOutput=[0]
  wires:
  Bus Selector1/2 -> Compute Errors/4(vl)  "<Xdot>"
  extraSpaceFlag/1 -> Compute Errors/5(lcFlag)
  Compute Errors/2(ev) -> Virtual Leader Following/2(ev), Mux/2
  Velocity Control/1(Out1) -> Chart/2(uVelControl)  "uVelControl"
  Bus Selector1/1 -> Compute Errors/3(xl)  "<X>"
  Chart/1(state) -> Transport Delay1/1
  Compute Errors/4(unsafeFlag) -> Terminator/1
  Chart/2(u) -> accel saturation/1
  Compute Errors/3("gap ") -> virtualGap/1
  Bus Selector/1 -> Compute Errors/1(xf)  "<X>"
  accel saturation/1 -> jerk saturation/1
  Bus Selector/2 -> Sum6/2, Compute Errors/2(vf)  "<Xdot>"
  Virtual Leader Following/1(u) -> Chart/3(uVehFoll)  "uVehFoll"
  Transport Delay1/1 -> Velocity Control/1(intReset)
  ego/1 -> Bus Selector/1
  Bus Selector/3 -> Virtual Leader Following/3(realInput)  "<u>"
  Compute Errors/1(eh) -> Mux/1, Virtual Leader Following/1(eh)  "eh"
  vMin/1 -> Sum6/1
  Mux/1 -> virtualErrors/1
  jerk saturation/1 -> u/1, Scope/1  "virtualFoll"
  virtualLeader/1 -> Bus Selector1/1
  Sum6/1 -> Chart/1(velDiff), Velocity Control/2(ev)

== system full_maneuver_platoon_new_strategy/p1/followerErrors ==
  ego : Inport
  follower : Inport  Port=2
  Bus Selector1 : BusSelector  OutputSignals=X,Xdot
  Bus Selector3 : BusSelector  OutputSignals=X,Xdot
  Mux : Mux  Inputs=2
  Sum3 : Sum  Inputs=-+|
  Terminator1 : Terminator
  gapToFollower : Subsystem
  errors : Outport
  wires:
  Mux/1 -> errors/1
  Bus Selector1/1 -> gapToFollower/3(xl)  "<X>"
  ego/1 -> Bus Selector1/1
  Bus Selector3/1 -> gapToFollower/1(xf)  "<X>"
  Bus Selector1/2 -> Sum3/2  "<Xdot>"
  gapToFollower/1(eh) -> Mux/1
  follower/1 -> Bus Selector3/1
  Bus Selector3/2 -> Sum3/1, gapToFollower/2(vf)  "<Xdot>"
  Sum3/1 -> Mux/2
  gapToFollower/2("gap ") -> Terminator1/1
